simulink model "Ghost_f34"  (Simulink 8.1)
settings: Solver=ode1  StartTime=0.0  StopTime=inf  FixedStep=Ts  MaxStep=1e-3  RelTol=1e-3
PostLoadFcn:
  | NREL_Mode=1; Ghost_init;
InitFcn:
  | NREL_Mode=1; Ghost_init;
values from neighbouring files (symbols this model uses):
  DER_REL = xlsread('DER_relay.xlsx')    [relay_settings_init.m]
  Ts = 100E-6    (= 0.0001)    [BANSHEE_init.m]    (also in Ghost_init.m)
undefined symbols (not defined in the file or in its folder): CBID, Feeder3_lib, Left, SM_UtilityService, SS_Feeder3, Stim, type, utility_service_lib, V
libraries: simulink x72, cables_lib x16, breaker_lib x14, transformer_lib x7, powerlib x7, rtlab x6, Load_lib x6, ssn_lib x4, artemis x2, PHIL_lib x2, rtio_generic_modbus x2, NREL_Diesel_Genset_lib x2
(part 3 of 3)

== system Ghost_f34/SC_ctrl/TestSequenceGen/uint32_2_uint16 ==
  In1 : Inport
  Data Type Conversion : DataTypeConversion  OutDataTypeStr=uint32
  Data Type Conversion1 : DataTypeConversion  OutDataTypeStr=double
  Data Type Conversion2 : DataTypeConversion  OutDataTypeStr=double
  Extract Bits : simulink/Logic and Bit Operations/Extract Bits  bitsToExtract=Upper half  numBits=8  bitIdxRange=[0 7]  outScalingMode=Treat bit field as an integer
  Extract Bits1 : simulink/Logic and Bit Operations/Extract Bits  bitsToExtract=Lower half  numBits=8  bitIdxRange=[0 7]  outScalingMode=Preserve fixed-point scaling
  Mux : Mux  Inputs=2
  Out1 : Outport
  wires:
  Mux/1 -> Out1/1
  Extract Bits/1 -> Data Type Conversion1/1
  In1/1 -> Data Type Conversion/1
  Data Type Conversion/1 -> Extract Bits1/1, Extract Bits/1
  Data Type Conversion2/1 -> Mux/1
  Data Type Conversion1/1 -> Mux/2
  Extract Bits1/1 -> Data Type Conversion2/1
